simulink model "problem1"  (R2020a)
settings: Solver=VariableStepAuto  StartTime=0.0  StopTime=10.0  RelTol=1e-3
model workspace (MAT data in the model file):
  K1 = Simulink.Parameter
  K1.Value = 50
  K1.DataType = 'auto'
  K1.Dimensions = [1 1]
  K12 = Simulink.Parameter
  K12.Value = 2000
  K12.DataType = 'auto'
  K12.Dimensions = [1 1]
  M1 = Simulink.Parameter
  M1.Value = 100
  M1.DataType = 'auto'
  M1.Dimensions = [1 1]
  M2 = Simulink.Parameter
  M2.Value = 50
  M2.DataType = 'auto'
  M2.Dimensions = [1 1]
  b = Simulink.Parameter
  b.Value = 50
  b.DataType = 'auto'
  b.Dimensions = [1 1]
settings Model: Creator=Riyansh  LastModifiedBy=Riyansh

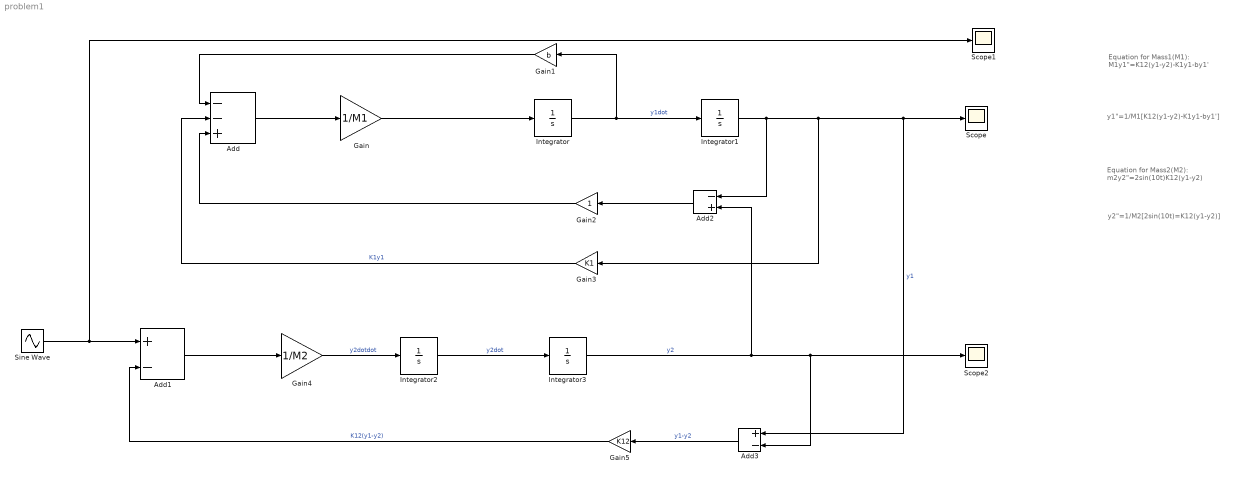
== system problem1 ==
  note: y2"=1/M2[2sin(10t)=K12(y1-y2)]
  note: Equation for Mass2(M2):
      | m2y2"=2sin(10t)K12(y1-y2)
  note: y1"=1/M1[K12(y1-y2)-K1y1-by1']
  note: Equation for Mass1(M1):
      | M1y1"=K12(y1-y2)-K1y1-by1'
  Add : Sum  Inputs=--+
  Add1 : Sum  Inputs=+-
  Add2 : Sum  Inputs=-+
  Add3 : Sum  Inputs=+-
  Gain : Gain  Gain=1/M1
  Gain1 : Gain  Gain=b
  Gain2 : Gain
  Gain3 : Gain  Gain=K1
  Gain4 : Gain  Gain=1/M2
  Gain5 : Gain  Gain=K12
  Integrator{,1..3} (4 alike) : Integrator
  Scope : Scope
  Scope1 : Scope
  Scope2 : Scope
  Sine Wave : Sin  SampleTime=0
  wires:
  Add3/1 -> Gain5/1  "y1-y2"
  Add/1 -> Gain/1
  Gain2/1 -> Add/3
  Integrator3/1 -> Add2/2, Add3/2, Scope2/1  "y2"
  Gain5/1 -> Add1/2  "K12(y1-y2)"
  Integrator2/1 -> Integrator3/1  "y2dot"
  Gain4/1 -> Integrator2/1  "y2dotdot"
  Sine Wave/1 -> Scope1/1, Add1/1
  Gain3/1 -> Add/2  "K1y1"
  Integrator/1 -> Gain1/1, Integrator1/1  "y1dot"
  Add2/1 -> Gain2/1
  Add1/1 -> Gain4/1
  Integrator1/1 -> Add2/1, Gain3/1, Add3/1, Scope/1  "y1"
  Gain/1 -> Integrator/1
  Gain1/1 -> Add/1
